simulink model "AW_test"  (R2015a)
settings: Solver=ode5  StartTime=0.0  StopTime=14  FixedStep=1e-4  RelTol=1e-3
values from neighbouring files (symbols this model uses):
  Ak = [-686.540167589 -2525.24249406 3003.88260074 -3376.17154505 -919.51585859 -329.995557257 0.554863416066 -1.08710235968 -676.651099981 -520.714667022 1.21590501094 -2.53862308337 ... (256 elements, 16x16)]    [controller.mat]    (also in main_matlab_step1.m = rlqg.A)
  Ap = Ap(nn-nnn+1:nn,nn-nnn+1:nn)    [main_matlab_step1.m]    (also in plant.mat = [-21.9168905393 -6329.30033318 0 0 0 0 0 0 0 0 0 0 ... (256 )
  Bk = [1.97719987834 -11.3684759745 -9.05802419262 10.0670713674 2.75617939968 0.986945919802 0.000704388812111 0.000546312859848 1.994467134 1.56925194637 -0.000623043221846 -0.000401188810085 ... (16 elements, 16x1)]    [controller.mat]    (also in main_matlab_step1.m = rlqg.B)
  Bp = B    [main_matlab_step1.m]    (also in plant.mat = [-0.0071257730068 0.00504040869295 -0.0390506420057 -0.06046)
  Ck = [222.229329693 -243.535885757 -178.555900893 231.804330898 -0.516735556885 1.68229660692 1.7803425243 2.91724348036 -1828.17787203 679.97679107 -124.670473614 -98.6387833172 ... (32 elements, 2x16)]    [controller.mat]    (also in main_matlab_step1.m = rlqg.C)
  Cp = C    [main_matlab_step1.m]    (also in plant.mat = [334.363840267 -876.077811885 -797.966835255 564.198773715 4)
  Dk = [0 0]    [controller.mat]    (also in main_matlab_step1.m = rlqg.D)
  GAMA1 = [632.493536651 -8005.74159669 -69.3665167828 19.5823393112 -9.76040872045 -23.0384394876 11.9275784463 -3.15541597641 0.122385837716 -4.14450623367 18.3136080323 -23.4723279238 ... (1024 elements, 32x32)]    [GAMA.mat]    (also in main_matlab_step3.m = GAMA(1:naw,1:naw); main_matlab_step3_test_for_delta.m = GAMA(1:naw,1:naw))
  GAMA2 = [-4782.5863493 -379.579729956 871.770358909 -16005.3713736 2315.69893844 3050.66018425 44018.5858622 2923.13409527 -12730.0351339 31543.5327603 124798.81398 9236.3459531 ... (64 elements, 32x2)]    [GAMA.mat]    (also in main_matlab_step3.m = GAMA(1:naw,naw+1:end); main_matlab_step3_test_for_delta.m = GAMA(1:naw,naw+1:end))
  GAMA3 = [-142176.534029 397971.567822 350192.145815 -243123.023205 -86010.5926036 -59580.3676994 789.491328664 -235.184944588 -8938.13884815 -28358.3447104 623.282245064 -137.692739798 ... (576 elements, 18x32)]    [GAMA.mat]    (also in main_matlab_step3.m = GAMA(naw+1:end,1:naw); main_matlab_step3_test_for_delta.m = GAMA(naw+1:end,1:naw))
  GAMA4 = [49.4859364222 -31.6458949911 -6.22548686543 -26.0992612391 -56.1557101672 28.4359299783 -349.624565767 592.989769394 -13.744884225 -6.27399322438 -377.012618092 739.985461751 ... (36 elements, 18x2)]    [GAMA.mat]    (also in main_matlab_step3.m = GAMA(naw+1:end,naw+1:end); main_matlab_step3_test_for_delta.m = GAMA(naw+1:end,naw+1:end))
  Hp = H    [main_matlab_step1.m]    (also in plant.mat = [0.306398734652 0.215313747918 0.40628061626 -0.589998589379)
  nc = nk    [main_matlab_step1.m]    (also in main_matlab_step3.m = nn; main_matlab_step3_test_for_delta.m = nn)
  nu = numel(Bpu)/np    [main_matlab_step1.m]    (also in main_matlab_step3.m = 2; main_matlab_step3_test_for_delta.m = 2)
libraries: simulink x1
settings Model: Creator=p4wp4w  LastModifiedBy=p4wp4w

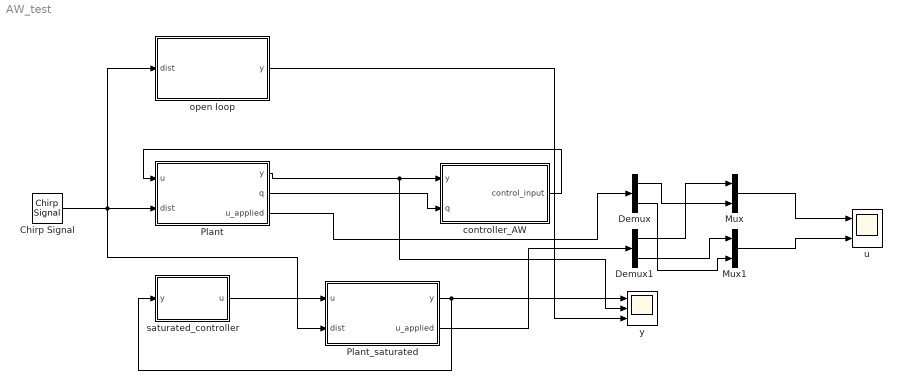
== system AW_test ==
  Chirp Signal : simulink/Sources/Chirp Signal  f1=0.1  T=14  f2=140
  Demux : Demux  Outputs=2
  Demux1 : Demux  Outputs=2
  Mux : Mux  Inputs=2
  Mux1 : Mux  Inputs=2
  Plant : Subsystem
  Plant_saturated : Subsystem
  controller_AW : Subsystem
  open loop : Subsystem
  "saturated_controller " : Subsystem
  u : Scope  NumInputPorts=2
      settings: YMin=-5~-5  YMax=5~5
  y : Scope  NumInputPorts=3
      settings: YMin=-5~-5~-5  YMax=5~5~5
  wires:
  Plant/1(y) -> y/2, controller_AW/1(y)
  Plant/2(q) -> controller_AW/2(q)
  controller_AW/1("control_input ") -> Plant/1(u)
  Chirp Signal/1 -> Plant_saturated/2(dist), open loop/1(dist), Plant/2(dist)
  "saturated_controller "/1(u) -> Plant_saturated/1(u)
  Plant_saturated/1(y) -> "saturated_controller "/1(y), y/1
  Demux1/1 -> Mux/1
  Demux/1 -> Mux/2
  Demux1/2 -> Mux1/1
  Demux/2 -> Mux1/2
  Mux/1 -> u/1
  Mux1/1 -> u/2
  Plant_saturated/2(u_applied) -> Demux1/1
  Plant/3(u_applied) -> Demux/1
  open loop/1(y) -> y/3

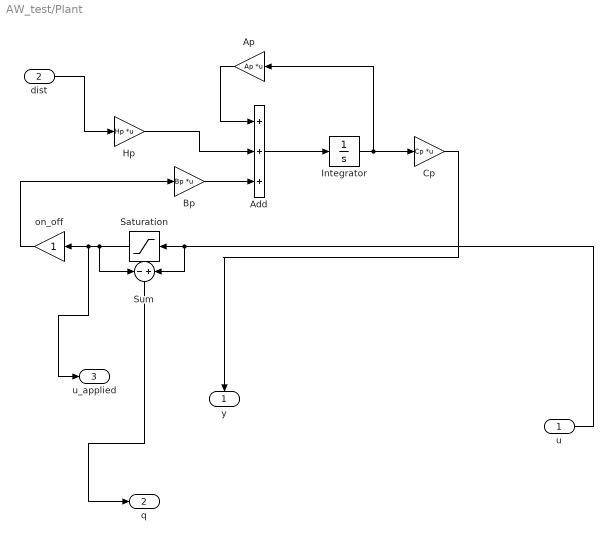
== system AW_test/Plant ==
  u : Inport
  dist : Inport  Port=2
  Add : Sum  Inputs=+++
  Ap : Gain  Gain=Ap  Multiplication=Matrix(K*u)
  Bp : Gain  Gain=Bp  Multiplication=Matrix(K*u)
  Cp : Gain  Gain=Cp  Multiplication=Matrix(K*u)
  Hp : Gain  Gain=Hp  Multiplication=Matrix(K*u)
  Integrator : Integrator
  Saturation : Saturate  UpperLimit=0.7  LowerLimit=-0.7
  Sum : Sum  Inputs=-|+
  on_off : Gain
  y : Outport
  q : Outport  Port=2
  u_applied : Outport  Port=3
  wires:
  Add/1 -> Integrator/1
  Cp/1 -> y/1
  Hp/1 -> Add/2
  on_off/1 -> Bp/1
  Integrator/1 -> Cp/1, Ap/1
  Saturation/1 -> Sum/1, u_applied/1, on_off/1
  Ap/1 -> Add/1
  u/1 -> Sum/2, Saturation/1
  Bp/1 -> Add/3
  Sum/1 -> q/1
  dist/1 -> Hp/1

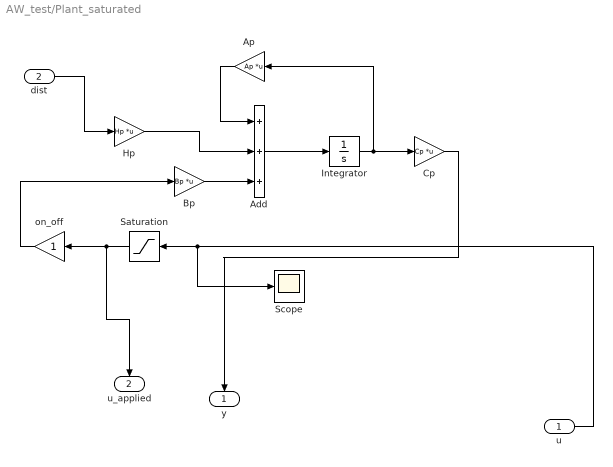
== system AW_test/Plant_saturated ==
  u : Inport
  dist : Inport  Port=2
  Add : Sum  Inputs=+++
  Ap : Gain  Gain=Ap  Multiplication=Matrix(K*u)
  Bp : Gain  Gain=Bp  Multiplication=Matrix(K*u)
  Cp : Gain  Gain=Cp  Multiplication=Matrix(K*u)
  Hp : Gain  Gain=Hp  Multiplication=Matrix(K*u)
  Integrator : Integrator
  Saturation : Saturate  UpperLimit=0.7  LowerLimit=-0.7
  Scope : Scope
      settings: YMin=-10  YMax=10  SaveName=ScopeData2
  on_off : Gain
  y : Outport
  u_applied : Outport  Port=2
  wires:
  dist/1 -> Hp/1
  Bp/1 -> Add/3
  u/1 -> Scope/1, Saturation/1
  Ap/1 -> Add/1
  Saturation/1 -> u_applied/1, on_off/1
  Integrator/1 -> Ap/1, Cp/1
  on_off/1 -> Bp/1
  Hp/1 -> Add/2
  Cp/1 -> y/1
  Add/1 -> Integrator/1

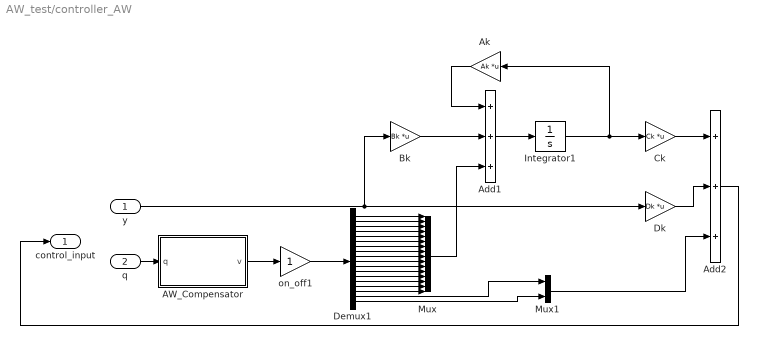
== system AW_test/controller_AW ==
  y : Inport
  q : Inport  Port=2
  AW_Compensator : Subsystem
  Add1 : Sum  Inputs=+++
  Add2 : Sum  Inputs=+++
  Ak : Gain  Gain=Ak  Multiplication=Matrix(K*u)
  Bk : Gain  Gain=Bk  Multiplication=Matrix(K*u)
  Ck : Gain  Gain=Ck  Multiplication=Matrix(K*u)
  Demux1 : Demux  Outputs=nc+nu
  Dk : Gain  Gain=Dk  Multiplication=Matrix(K*u)
  Integrator1 : Integrator
  Mux : Mux  Inputs=nc
  Mux1 : Mux  Inputs=nu
  on_off1 : Gain
  "control_input " : Outport
  wires:
  Ck/1 -> Add2/1
  Add1/1 -> Integrator1/1
  Ak/1 -> Add1/1
  AW_Compensator/1(v) -> on_off1/1
  Bk/1 -> Add1/2
  Integrator1/1 -> Ck/1, Ak/1
  Dk/1 -> Add2/2
  on_off1/1 -> Demux1/1
  Mux1/1 -> Add2/3
  Mux/1 -> Add1/3
  y/1 -> Bk/1, Dk/1
  q/1 -> AW_Compensator/1(q)
  Add2/1 -> "control_input "/1
  Demux1/10 -> Mux/10
  Demux1/9 -> Mux/9
  Demux1/12 -> Mux/12
  Demux1/13 -> Mux/13
  Demux1/11 -> Mux/11
  Demux1/15 -> Mux/15
  Demux1/16 -> Mux/16
  Demux1/14 -> Mux/14
  Demux1/1 -> Mux/1
  Demux1/2 -> Mux/2
  Demux1/3 -> Mux/3
  Demux1/4 -> Mux/4
  Demux1/8 -> Mux/8
  Demux1/6 -> Mux/6
  Demux1/5 -> Mux/5
  Demux1/7 -> Mux/7
  Demux1/17 -> Mux1/1
  Demux1/18 -> Mux1/2

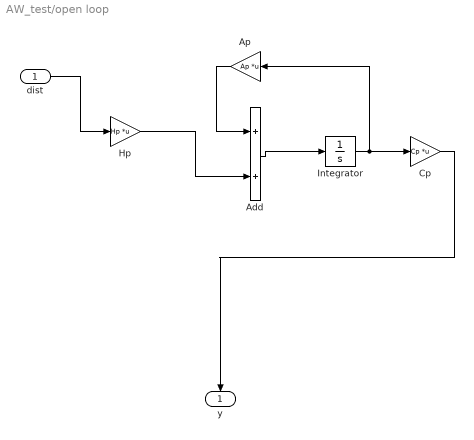
== system AW_test/open loop ==
  dist : Inport
  Add : Sum
  Ap : Gain  Gain=Ap  Multiplication=Matrix(K*u)
  Cp : Gain  Gain=Cp  Multiplication=Matrix(K*u)
  Hp : Gain  Gain=Hp  Multiplication=Matrix(K*u)
  Integrator : Integrator
  y : Outport
  wires:
  dist/1 -> Hp/1
  Ap/1 -> Add/1
  Integrator/1 -> Ap/1, Cp/1
  Hp/1 -> Add/2
  Cp/1 -> y/1
  Add/1 -> Integrator/1

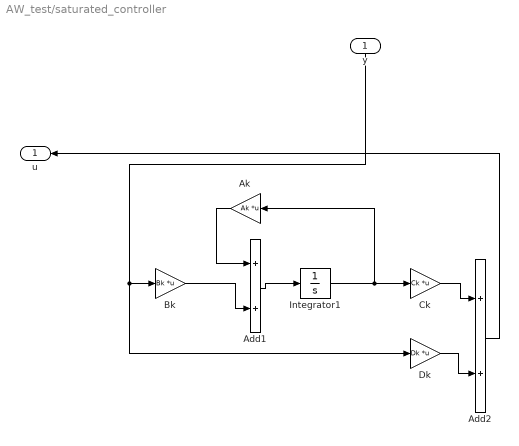
== system AW_test/saturated_controller  ==
  y : Inport
  Add1 : Sum
  Add2 : Sum
  Ak : Gain  Gain=Ak  Multiplication=Matrix(K*u)
  Bk : Gain  Gain=Bk  Multiplication=Matrix(K*u)
  Ck : Gain  Gain=Ck  Multiplication=Matrix(K*u)
  Dk : Gain  Gain=Dk  Multiplication=Matrix(K*u)
  Integrator1 : Integrator
  u : Outport
  wires:
  Bk/1 -> Add1/2
  Add1/1 -> Integrator1/1
  Ck/1 -> Add2/1
  Dk/1 -> Add2/2
  Integrator1/1 -> Ck/1, Ak/1
  Add2/1 -> u/1
  Ak/1 -> Add1/1
  y/1 -> Bk/1, Dk/1

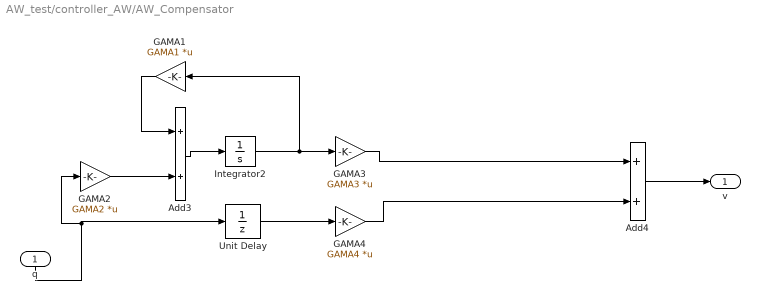
== system AW_test/controller_AW/AW_Compensator ==
  q : Inport
  Add3 : Sum
  Add4 : Sum
  GAMA1 : Gain  Gain=GAMA1  Multiplication=Matrix(K*u)
  GAMA2 : Gain  Gain=GAMA2  Multiplication=Matrix(K*u)
  GAMA3 : Gain  Gain=GAMA3  Multiplication=Matrix(K*u)
  GAMA4 : Gain  Gain=GAMA4  Multiplication=Matrix(K*u)
  Integrator2 : Integrator
  Unit Delay : UnitDelay  SampleTime=-1
  v : Outport
  wires:
  Add3/1 -> Integrator2/1
  GAMA3/1 -> Add4/1
  GAMA1/1 -> Add3/1
  Integrator2/1 -> GAMA3/1, GAMA1/1
  GAMA2/1 -> Add3/2
  GAMA4/1 -> Add4/2
  Add4/1 -> v/1
  q/1 -> Unit Delay/1, GAMA2/1
  Unit Delay/1 -> GAMA4/1
